simulink model "task3"  (R2023a)
settings: Solver=VariableStepAuto  StartTime=0.0  StopTime=10.0  RelTol=1e-8
settings Model: Creator=user  LastModifiedBy=user

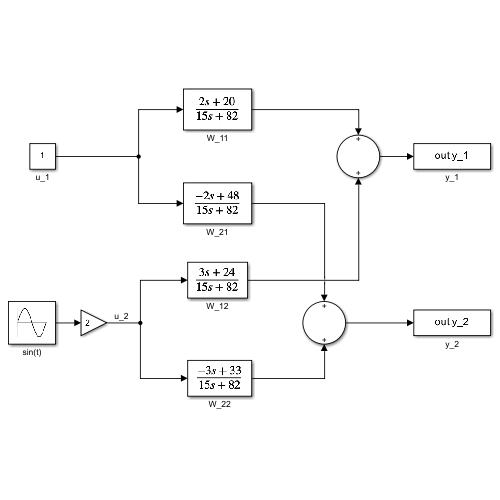
[thumbnail: Simulink's stored preview of the top-level diagram]
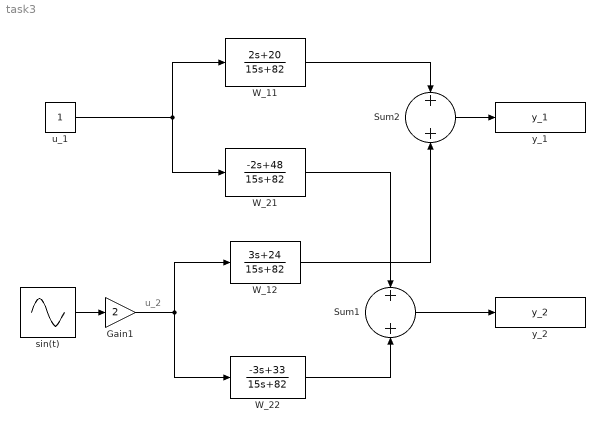
== system task3 ==
  note: u_2
  Gain1 : Gain  Gain=2
  Sum1 : Sum
  Sum2 : Sum
  W_11 : TransferFcn  Numerator=[2 20]  Denominator=[15 82]
  W_12 : TransferFcn  Numerator=[3 24]  Denominator=[15 82]
  W_21 : TransferFcn  Numerator=[-2 48]  Denominator=[15 82]
  W_22 : TransferFcn  Numerator=[-3 33]  Denominator=[15 82]
  sin(t) : Sin  SampleTime=0
  u_1 : Constant
  y_1 : ToWorkspace  VariableName=y_1  SaveFormat=Timeseries  SampleTime=-1
  y_2 : ToWorkspace  VariableName=y_2  SaveFormat=Timeseries  SampleTime=-1
  wires:
  u_1/1 -> W_21/1, W_11/1
  Gain1/1 -> W_22/1, W_12/1
  Sum2/1 -> y_1/1
  Sum1/1 -> y_2/1
  W_11/1 -> Sum2/1
  W_12/1 -> Sum2/2
  W_21/1 -> Sum1/1
  W_22/1 -> Sum1/2
  sin(t)/1 -> Gain1/1
